simulink model "PV_GHI_System_Mezoo_3"  (R2024b)
settings: Solver=ode3  StartTime=0.0  StopTime=259200  FixedStep=60  RelTol=1e-3
InitFcn:
  | % --- تحديث كود تهيئة السيمولينك (InitFcn) ---
  | disp('>>> 1. جاري تحضير العقل (Loading Neural Network)...');
  | 
  | % تحديد المسار الصحيح للمشروع الحالي
  | Project_Path = 'D:\Project\Agent Vini';
  | if exist(Project_Path, 'dir')
  |     addpath(Project_Path);
  | end
  | 
  | % اسم الملف الجديد (تأكد أن هذا هو الاسم الموجود عندك في المجلد)
  | Model_File = 'Lightweight_Model.mat';
  | 
  | % محاولة التحميل
  | if exist(Model_File, 'file')
  |     FileData = load(Model_File);
  |     disp(['✅ تم تحميل الملف: ' Model_File]);
  | else
  |     % محاولة البحث في المجلد القديم كحل مؤقت لو الملف لم ينقل
  |     Old_Path = 'D:\Project\Agent 13';
  |     if exist(fullfile(Old_Path, 'PI_HybridNet.mat'), 'file')
  |         addpath(Old_Path);
  |         FileData = load('PI_HybridNet.mat');
  |         warning('⚠️ تم تحميل الملف القديم من Agent 13 لأن الجديد غير موجود!');
  |     else
  |         error('❌ لم يتم العثور على ملف النموذج (لا الجديد ولا القديم)!');
  |     end
  | end
  | 
  | % استخراج الشبكة (سواء كان اسمها net أو net_best أو net_light)
  | if isfield(FileData, 'net_light')
  |     net_ready = FileData.net_light;
  | elseif isfield(FileData, 'net')
  |     net_ready = FileData.net;
  | elseif isfield(FileData, 'net_best')
  |     net_ready = FileData.net_best;
  | else
  |     % ربما المتغير نفسه هو الشبكة
  |     VarNames = fieldnames(FileData);
  |     net_ready = FileData.(VarNames{1});
  | end
  | 
  | disp('>>> 2. العقل جاهز في الذاكرة باسم: net_ready');
undefined symbols (not defined in the file or in its folder): A, History_Day1, History_Day2, History_Day3, Max_Tank, mu_X, mu_Y, sig_X, sig_Y
libraries: mpclib x1
settings Model: Creator=moham  LastModifiedBy=moham
settings DebuggingCC: AlgebraicLoopMsg=none

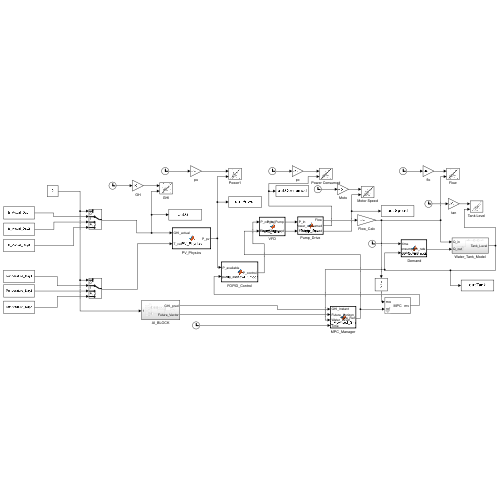
[thumbnail: Simulink's stored preview of the top-level diagram]
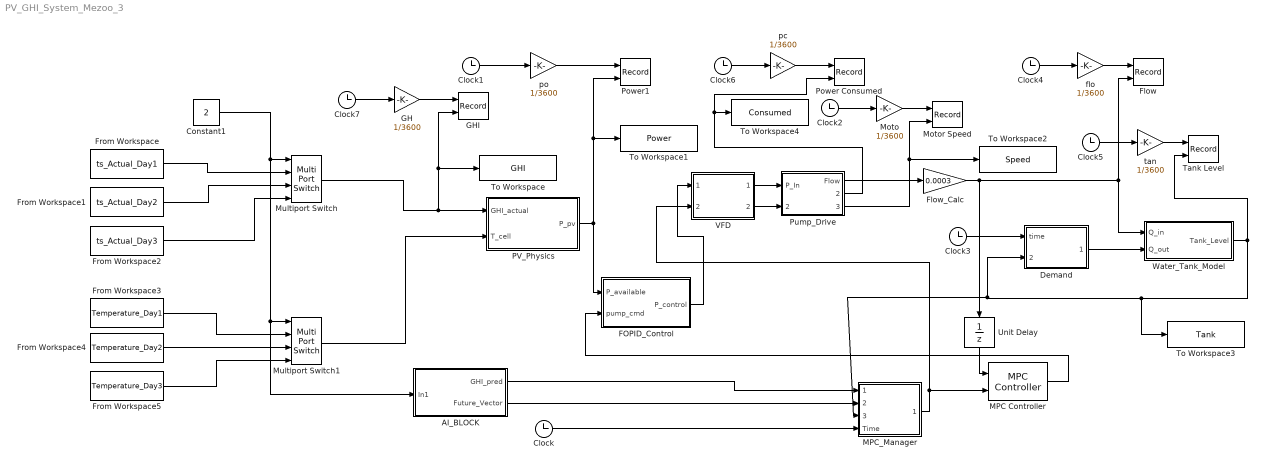
== system PV_GHI_System_Mezoo_3 ==
  " Demand" : MATLAB Function  TreatAsAtomicUnit=on
  AI_BLOCK : Subsystem
  Clock{,1..7} (8 alike) : Clock
  Constant1 : Constant  Value=2
  FOPID_Control : MATLAB Function  TreatAsAtomicUnit=on
  Flow : Record  FileSettingsInternal="{\"entries\":[{\"content\":{\"excelSettings\":{\"content\":{},\"type\":\"Streamout.ExcelSettings\"}},\"type\":\"Streamout.FileSettingStorage\",\"uuid\":\"\"}],\"packageUris\":[\"http:\\/\\/schema.mathworks.com\\/mf0\\/streamout_blocks\\/R2020a\"],\"version\":\"1.0\"}"  Layout=[1 1]  SignalsInternal="{\"entries\":[{\"content\":{\"signals\":[{\"content\":{\"blockPath\":[],\"dimensions\":[1],\"domain\":\"\",\"lineColor\":\"#b746ff\",\"lineWidth\":2,\"port\":1,\"sid\":[\"\"],\"signalID\":1,\"signalName\":\"flo\"},\"type\":\"RecordBlkView.Signal\",\"uuid\":\"\"},{\"content\":{\"blockPath\":[],\"dimensions\":[1],\"domain\":\"\",\"lineColor\":\"#64d413\",\"lineWidth\":2,\"port\":2,\"sid\":[\"\"],\"signalID\":2,\"signalName\":\"Flow_Calc\"},\"type\":\"RecordBlkView.Signal\",\"uuid\":\"\"}]},\"type\":\"RecordBlkView.InputSignals\",\"uuid\":\"\"}],\"packageUris\":[\"http:\\/\\/schema.mathworks.com\\/mf0\\/streamout_blocks\\/R2020a\"],\"version\":\"1.0\"}"  VisualizationBindings="{\"xyplotplugin\":{\"info\":[{\"series\":[],\"subplotID\":1}]}}"  CompatibilityTag=XY
  Flow_Calc : Gain  Gain=0.0003
  From Workspace : FromWorkspace  VariableName=ts_Actual_Day1
  From Workspace1 : FromWorkspace  VariableName=ts_Actual_Day2
  From Workspace2 : FromWorkspace  VariableName=ts_Actual_Day3
  From Workspace3 : FromWorkspace  VariableName=Temperature_Day1
  From Workspace4 : FromWorkspace  VariableName=Temperature_Day2
  From Workspace5 : FromWorkspace  VariableName=Temperature_Day3
  GH : Gain  Gain=1/3600
  GHI : Record  FileSettingsInternal="{\"entries\":[{\"content\":{\"excelSettings\":{\"content\":{},\"type\":\"Streamout.ExcelSettings\"}},\"type\":\"Streamout.FileSettingStorage\",\"uuid\":\"\"}],\"packageUris\":[\"http:\\/\\/schema.mathworks.com\\/mf0\\/streamout_blocks\\/R2020a\"],\"version\":\"1.0\"}"  Layout=[1 1]  SignalsInternal="{\"entries\":[{\"content\":{\"signals\":[{\"content\":{\"blockPath\":[],\"dimensions\":[1],\"domain\":\"\",\"lineColor\":\"#ff13a6\",\"lineWidth\":2,\"plots\":[ 1 ],\"port\":1,\"sid\":[\"\"],\"signalID\":1,\"signalName\":\"GH\"},\"type\":\"RecordBlkView.Signal\",\"uuid\":\"\"},{\"content\":{\"blockPath\":[],\"dimensions\":[1],\"domain\":\"\",\"lineColor\":\"#fe330a\",\"lineWidth\":2,\"plots\":[ 1 ],\"port\":2,\"sid\":[\"\"],\"signalID\":2,\"signalName\":\"Multiport\\nSwitch\"},\"type\":\"RecordBlkView.Signal\",\"uuid\":\"\"}]},\"type\":\"RecordBlkView.InputSignals\",\"uuid\":\"\"}],\"packageUris\":[\"http:\\/\\/schema.mathworks.com\\/mf0\\/streamout_blocks\\/R2020a\"],\"version\":\"1.0\"}"  VisualizationBindings="{\"xyplotplugin\":{\"info\":[{\"series\":[{\"bindingParametersList\":[{\"parameter\":\"X-Axis\",\"signalID\":1,\"signalName\":\"GH\"},{\"parameter\":\"Y-Axis\",\"signalID\":2,\"signalName\":\"Multiport\\nSwitch\"}],\"seriesID\":0}],\"subplotID\":1}]}}"  CompatibilityTag=XY
  MPC Controller : mpclib/MPC Controller  SCDEnableBlockLinearizationSpecification=on  mpcobj=MPC_Obj  is_multiple=0  enable_value=0  return_u0=off  updateMPCinCallerWorkspace=on  md_inport=off  mv_inport=off  uref_inport=off  return_cost=off  return_mvseq=off  return_qpstatus=off  return_xseq=off  return_state=off  return_ovseq=off  state_inport=off  umin_inport=off  umax_inport=off  ymin_inport=off  ymax_inport=off  cc_inport=off  ywt_inport=off  uwt_inport=off  duwt_inport=off  rhoeps_inport=off  pm_inport=off  MaximumP=10  HorizonChoice=FixedHorizon  n_ts=60  n_p=300  n_mv=1  n_md=0  n_ud=0  n_mo=1  n_uo=0  BlockDataType=double  SampleTimeInherited=off  switch_inport=off
  MPC_Manager : MATLAB Function  TreatAsAtomicUnit=on
  Moto : Gain  Gain=1/3600
  Motor Speed : Record  FileSettingsInternal="{\"entries\":[{\"content\":{\"excelSettings\":{\"content\":{},\"type\":\"Streamout.ExcelSettings\"}},\"type\":\"Streamout.FileSettingStorage\",\"uuid\":\"\"}],\"packageUris\":[\"http:\\/\\/schema.mathworks.com\\/mf0\\/streamout_blocks\\/R2020a\"],\"version\":\"1.0\"}"  Layout=[1 1]  SignalsInternal="{\"entries\":[{\"content\":{\"signals\":[{\"content\":{\"blockPath\":[],\"dimensions\":[1],\"domain\":\"\",\"lineColor\":\"#139fff\",\"lineWidth\":2,\"plots\":[ 1 ],\"port\":1,\"sid\":[\"\"],\"signalID\":1,\"signalName\":\"Moto\"},\"type\":\"RecordBlkView.Signal\",\"uuid\":\"\"},{\"content\":{\"blockPath\":[],\"dimensions\":[1],\"domain\":\"\",\"lineColor\":\"#ff6929\",\"lineWidth\":2,\"plots\":[ 1 ],\"port\":2,\"sid\":[\"\"],\"signalID\":2,\"signalName\":\"Pump_Drive:3\"},\"type\":\"RecordBlkView.Signal\",\"uuid\":\"\"}]},\"type\":\"RecordBlkView.InputSignals\",\"uuid\":\"\"}],\"packageUris\":[\"http:\\/\\/schema.mathworks.com\\/mf0\\/streamout_blocks\\/R2020a\"],\"version\":\"1.0\"}"  VisualizationBindings="{\"xyplotplugin\":{\"info\":[{\"series\":[{\"bindingParametersList\":[{\"parameter\":\"X-Axis\",\"signalID\":1,\"signalName\":\"Moto\"},{\"parameter\":\"Y-Axis\",\"signalID\":2,\"signalName\":\"Pump_Drive:3\"}],\"seriesID\":0}],\"subplotID\":1}]}}"  CompatibilityTag=XY
  Multiport Switch : MultiPortSwitch  DataPortOrder=Zero-based contiguous  DiagnosticForDefault=Warning  zeroidx=on  SaturateOnIntegerOverflow=off  InputSameDT=off
  Multiport Switch1 : MultiPortSwitch  DataPortOrder=Zero-based contiguous  DiagnosticForDefault=Warning  zeroidx=on  SaturateOnIntegerOverflow=off  InputSameDT=off
  PV_Physics : MATLAB Function  TreatAsAtomicUnit=on
  Power Consumed : Record  FileSettingsInternal="{\"entries\":[{\"content\":{\"excelSettings\":{\"content\":{},\"type\":\"Streamout.ExcelSettings\"}},\"type\":\"Streamout.FileSettingStorage\",\"uuid\":\"\"}],\"packageUris\":[\"http:\\/\\/schema.mathworks.com\\/mf0\\/streamout_blocks\\/R2020a\"],\"version\":\"1.0\"}"  Layout=[1 1]  SignalsInternal="{\"entries\":[{\"content\":{\"signals\":[{\"content\":{\"blockPath\":[],\"dimensions\":[1],\"domain\":\"\",\"lineColor\":\"#d95319\",\"lineWidth\":2,\"port\":1,\"sid\":[\"\"],\"signalID\":1,\"signalName\":\"pc\"},\"type\":\"RecordBlkView.Signal\",\"uuid\":\"\"},{\"content\":{\"blockPath\":[],\"dimensions\":[1],\"domain\":\"\",\"lineColor\":\"#edb120\",\"lineWidth\":2,\"port\":2,\"sid\":[\"\"],\"signalID\":2,\"signalName\":\"Pump_Drive:2\"},\"type\":\"RecordBlkView.Signal\",\"uuid\":\"\"}]},\"type\":\"RecordBlkView.InputSignals\",\"uuid\":\"\"}],\"packageUris\":[\"http:\\/\\/schema.mathworks.com\\/mf0\\/streamout_blocks\\/R2020a\"],\"version\":\"1.0\"}"  VisualizationBindings="{\"xyplotplugin\":{\"info\":[{\"series\":[],\"subplotID\":1}]}}"  CompatibilityTag=XY
  Power1 : Record  FileSettingsInternal="{\"entries\":[{\"content\":{\"excelSettings\":{\"content\":{},\"type\":\"Streamout.ExcelSettings\"}},\"type\":\"Streamout.FileSettingStorage\",\"uuid\":\"\"}],\"packageUris\":[\"http:\\/\\/schema.mathworks.com\\/mf0\\/streamout_blocks\\/R2020a\"],\"version\":\"1.0\"}"  Layout=[1 1]  SignalsInternal="{\"entries\":[{\"content\":{\"signals\":[{\"content\":{\"blockPath\":[],\"dimensions\":[1],\"domain\":\"\",\"lineColor\":\"#7e2f8e\",\"lineWidth\":2,\"port\":1,\"sid\":[\"\"],\"signalID\":1,\"signalName\":\"po\"},\"type\":\"RecordBlkView.Signal\",\"uuid\":\"\"},{\"content\":{\"blockPath\":[],\"dimensions\":[1],\"domain\":\"\",\"lineColor\":\"#77ac30\",\"lineWidth\":2,\"port\":2,\"sid\":[\"\"],\"signalID\":2,\"signalName\":\"PV_Physics\"},\"type\":\"RecordBlkView.Signal\",\"uuid\":\"\"}]},\"type\":\"RecordBlkView.InputSignals\",\"uuid\":\"\"}],\"packageUris\":[\"http:\\/\\/schema.mathworks.com\\/mf0\\/streamout_blocks\\/R2020a\"],\"version\":\"1.0\"}"  VisualizationBindings="{\"xyplotplugin\":{\"info\":[{\"series\":[],\"subplotID\":1}]}}"  CompatibilityTag=XY
  Pump_Drive : MATLAB Function  TreatAsAtomicUnit=on
  Tank Level : Record  FileSettingsInternal="{\"entries\":[{\"content\":{\"excelSettings\":{\"content\":{},\"type\":\"Streamout.ExcelSettings\"}},\"type\":\"Streamout.FileSettingStorage\",\"uuid\":\"\"}],\"packageUris\":[\"http:\\/\\/schema.mathworks.com\\/mf0\\/streamout_blocks\\/R2020a\"],\"version\":\"1.0\"}"  Layout=[1 1]  SignalsInternal="{\"entries\":[{\"content\":{\"signals\":[{\"content\":{\"blockPath\":[],\"dimensions\":[1],\"domain\":\"\",\"lineColor\":\"#4dbeee\",\"lineWidth\":2,\"plots\":[ 1 ],\"port\":1,\"sid\":[\"\"],\"signalID\":1,\"signalName\":\"tan\"},\"type\":\"RecordBlkView.Signal\",\"uuid\":\"\"},{\"content\":{\"blockPath\":[],\"dimensions\":[1],\"domain\":\"\",\"lineColor\":\"#a2142f\",\"lineWidth\":2,\"plots\":[ 1 ],\"port\":2,\"sid\":[\"\"],\"signalID\":2,\"signalName\":\"Water_Tank_Model\"},\"type\":\"RecordBlkView.Signal\",\"uuid\":\"\"}]},\"type\":\"RecordBlkView.InputSignals\",\"uuid\":\"\"}],\"packageUris\":[\"http:\\/\\/schema.mathworks.com\\/mf0\\/streamout_blocks\\/R2020a\"],\"version\":\"1.0\"}"  VisualizationBindings="{\"xyplotplugin\":{\"info\":[{\"series\":[{\"bindingParametersList\":[{\"parameter\":\"X-Axis\",\"signalID\":1,\"signalName\":\"tan\"},{\"parameter\":\"Y-Axis\",\"signalID\":2,\"signalName\":\"Water_Tank_Model\"}],\"seriesID\":0}],\"subplotID\":1}]}}"  CompatibilityTag=XY
  To Workspace : ToWorkspace  VariableName=GHI  SaveFormat=Timeseries  SampleTime=-1
  To Workspace1 : ToWorkspace  VariableName=Power  SaveFormat=Timeseries  SampleTime=-1
  To Workspace2 : ToWorkspace  VariableName=Speed  SaveFormat=Timeseries  SampleTime=-1
  To Workspace3 : ToWorkspace  VariableName=Tank  SaveFormat=Timeseries  SampleTime=-1
  To Workspace4 : ToWorkspace  VariableName=Consumed  SaveFormat=Timeseries  SampleTime=-1
  Unit Delay : UnitDelay  SampleTime=60  HasFrameUpgradeWarning=on
  VFD : MATLAB Function  TreatAsAtomicUnit=on
  Water_Tank_Model : Subsystem
  flo : Gain  Gain=1/3600
  pc : Gain  Gain=1/3600
  po : Gain  Gain=1/3600
  tan : Gain  Gain=1/3600
  wires:
  Water_Tank_Model/1(Tank_Level) -> To Workspace3/1, MPC_Manager/3(Water_Level), " Demand"/2(water_level), Tank Level/2
  Flow_Calc/1 -> Unit Delay/1, Flow/2, Water_Tank_Model/1(Q_in)
  Pump_Drive/1(Flow) -> Flow_Calc/1
  Pump_Drive/2(Power_consumed) -> To Workspace4/1, Power Consumed/2
  Pump_Drive/3(Motor_Speed) -> To Workspace2/1, Motor Speed/2
  Clock1/1 -> po/1
  po/1 -> Power1/1
  flo/1 -> Flow/1
  Clock4/1 -> flo/1
  Clock5/1 -> tan/1
  tan/1 -> Tank Level/1
  Clock2/1 -> Moto/1
  Moto/1 -> Motor Speed/1
  Clock6/1 -> pc/1
  pc/1 -> Power Consumed/1
  Clock7/1 -> GH/1
  GH/1 -> GHI/1
  PV_Physics/1(P_pv) -> To Workspace1/1, Power1/2, FOPID_Control/1(P_available)
  Multiport Switch/1 -> To Workspace/1, GHI/2, PV_Physics/1(GHI_actual)
  Constant1/1 -> Multiport Switch1/1, AI_BLOCK/1(In1), Multiport Switch/1
  From Workspace/1 -> Multiport Switch/2
  From Workspace1/1 -> Multiport Switch/3
  From Workspace2/1 -> Multiport Switch/4
  " Demand"/1(consumption_rate) -> Water_Tank_Model/2(Q_out)
  Clock3/1 -> " Demand"/1(time)
  FOPID_Control/1(P_control) -> VFD/1(P_control)
  VFD/1(P_to_Pump) -> Pump_Drive/1(P_In)
  VFD/2(Flow_Command) -> Pump_Drive/2(Flow_In)
  MPC_Manager/1(Flow_Ref) -> VFD/2(target_flow), MPC Controller/2
  MPC Controller/1 -> FOPID_Control/2(pump_cmd)
  Unit Delay/1 -> MPC Controller/1
  Clock/1 -> MPC_Manager/4(Time)
  AI_BLOCK/1(GHI_pred) -> MPC_Manager/1(GHI_Instant)
  From Workspace4/1 -> Multiport Switch1/3
  From Workspace3/1 -> Multiport Switch1/2
  From Workspace5/1 -> Multiport Switch1/4
  Multiport Switch1/1 -> PV_Physics/2(T_cell)
  AI_BLOCK/2(Future_Vector) -> MPC_Manager/2(Future_Horizon)

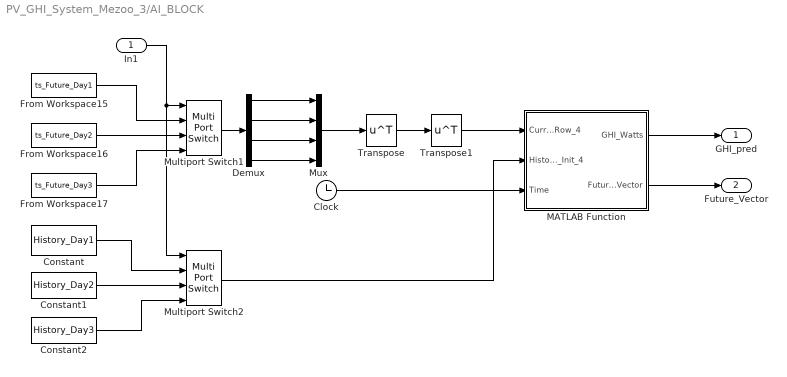
== system PV_GHI_System_Mezoo_3/AI_BLOCK ==
  In1 : Inport
  Clock : Clock
  Constant : Constant  Value=History_Day1
  Constant1 : Constant  Value=History_Day2
  Constant2 : Constant  Value=History_Day3
  Demux : Demux
  From Workspace15 : FromWorkspace  VariableName=ts_Future_Day1
  From Workspace16 : FromWorkspace  VariableName=ts_Future_Day2
  From Workspace17 : FromWorkspace  VariableName=ts_Future_Day3
  MATLAB Function : MATLAB Function  TreatAsAtomicUnit=on
  Multiport Switch1 : MultiPortSwitch  DataPortOrder=Zero-based contiguous  DiagnosticForDefault=Warning  zeroidx=on  SaturateOnIntegerOverflow=off  InputSameDT=off
  Multiport Switch2 : MultiPortSwitch  DataPortOrder=Zero-based contiguous  DiagnosticForDefault=Warning  zeroidx=on  SaturateOnIntegerOverflow=off  InputSameDT=off
  Mux : Mux
  Transpose : Math  Operator=transpose
  Transpose1 : Math  Operator=transpose
  GHI_pred : Outport
  Future_Vector : Outport  Port=2
  wires:
  From Workspace16/1 -> Multiport Switch1/3
  From Workspace17/1 -> Multiport Switch1/4
  From Workspace15/1 -> Multiport Switch1/2
  In1/1 -> Multiport Switch2/1, Multiport Switch1/1
  Multiport Switch1/1 -> Demux/1
  MATLAB Function/1(GHI_Watts) -> GHI_pred/1
  Mux/1 -> Transpose/1
  Constant/1 -> Multiport Switch2/2
  Constant1/1 -> Multiport Switch2/3
  Constant2/1 -> Multiport Switch2/4
  Multiport Switch2/1 -> MATLAB Function/2(History_Init_4)
  Transpose/1 -> Transpose1/1
  Transpose1/1 -> MATLAB Function/1(Current_Row_4)
  Clock/1 -> MATLAB Function/3(Time)
  Demux/1 -> Mux/1
  Demux/2 -> Mux/2
  Demux/3 -> Mux/3
  Demux/4 -> Mux/4
  MATLAB Function/2(Future_Vector) -> Future_Vector/1

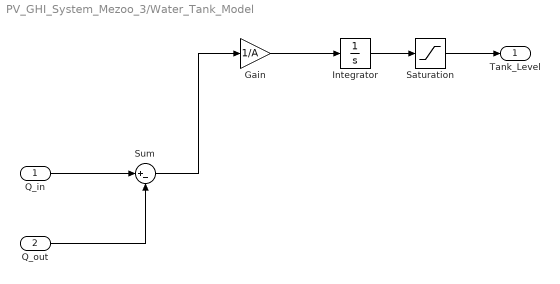
== system PV_GHI_System_Mezoo_3/Water_Tank_Model ==
  Q_in : Inport
  Q_out : Inport  Port=2
  Gain : Gain  Gain=1/A
  Integrator : Integrator  InitialCondition=4
  Saturation : Saturate  UpperLimit=Max_Tank  LowerLimit=0
  Sum : Sum  Inputs=|+-
  Tank_Level : Outport
  wires:
  Q_in/1 -> Sum/1
  Sum/1 -> Gain/1
  Integrator/1 -> Saturation/1
  Saturation/1 -> Tank_Level/1
  Q_out/1 -> Sum/2
  Gain/1 -> Integrator/1

== matlab function PV_GHI_System_Mezoo_3/FOPID_Control ==
  settings: updateMethod=DISCRETE
  data: P_available input; P_control output; pump_cmd input

function P_control = FOPID_Control_Smooth(P_available, pump_cmd)

%% FOPID Parameters (تم تنعيمها قليلاً لتقليل العدوانية)
Kp = 1.0;   % قللناها من 1.2 لتقليل رد الفعل العنيف
Ki = 0.5;   % التكامل يسبب تذبذباً إذا كان عالياً، 0.5 كافية جداً
Kd = 0.01;  % زدنا التفاضل قليلاً لامتصاص الصدمات
lambda = 0.9;
mu     = 0.7;

%% Persistent states (ذاكرة)
persistent e_int e_prev prev_P_out is_running
if isempty(e_int)
    e_int  = 0;
    e_prev = 0;
    prev_P_out = 0;   % لتنعيم الخرج
    is_running = 0;   % حالة التشغيل (للسماحية)
end

%% ===============================
%% 1. إيقاف فوري للأوامر الصفرية
%% ===============================
if pump_cmd == 0
    e_int = 0;
    e_prev = 0;
    prev_P_out = 0;
    is_running = 0;
    P_control = 0;
    return;
end

%% Reference
P_ref = pump_cmd * P_available;

%% Error definition
e = P_ref;

%% Fractional Integral
e_int = e_int + sign(e) * abs(e)^lambda;
% حماية من التراكم (Windup)
e_int = max(-5000, min(5000, e_int));

%% Fractional Derivative
de = sign(e - e_prev) * abs(e - e_prev)^mu;
e_prev = e;

%% FOPID Law
P_raw = Kp*e + Ki*e_int + Kd*de;

%% Saturation (الحدود الفيزيائية)
P_raw = max(0, min(P_available, P_raw));

%% ===============================
%% 2. نظام السماحية (Hysteresis) - مانع التذبذب رقم 1
%% ===============================
% بدلاً من رقم واحد (2200)، نستخدم رقمين:
START_THRESH = 2400;  % لا تبدأ إلا لو الطاقة قوية
STOP_THRESH  = 2000;  % لا تقف إلا لو الطاقة ضعفت جداً

if is_running == 0
    if P_raw > START_THRESH
        is_running = 1;
    else
        is_running = 0;
    end
else
    if P_raw < STOP_THRESH
        is_running = 0;
    else
        is_running = 1;
    end
end

if is_running == 0
    Target_P = 0;
    e_int = 0; % تصفير التكامل عند التوقف لمنع القفزة عند العودة
else
    Target_P = P_raw;
end

%% ===============================
%% 3. منع الصدمات (Rate Limiter) - مانع التذبذب رقم 2
%% ===============================
% نمنع الطاقة من التغير بأكثر من 100 واط في الخطوة الواحدة
% هذا يجعل صوت الموتور ناعماً ويمنع "النتعة"
MAX_RATE = 150; 

delta = Target_P - prev_P_out;

if abs(delta) > MAX_RATE
    P_control = prev_P_out + sign(delta) * MAX_RATE;
else
    P_control = Target_P;
end

% تحديث الذاكرة
prev_P_out = P_control;

end

== matlab function PV_GHI_System_Mezoo_3/ Demand ==
  data: time input; consumption_rate output; water_level input
function consumption_rate = Crop_Consumption(time, water_level)
%% =========================================================
%%  استهلاك الزراعة الواقعي (5 فدان - ري بالتنقيط - أم درمان)
%%  الاحتياج اليومي: 100,000 لتر (100 متر مكعب)
%%  نظام الري: يعمل 12 ساعة (من 6 ص إلى 6 م)
%% =========================================================

%% التوقيت
hour = mod(time/3600, 24);
DAY_START = 6; 
DAY_END = 18;

%% حساب المعدل (Base Rate)
% الهدف: 100 متر مكعب خلال 12 ساعة تشغيل
% المعادلة: 100 / (12 ساعة * 3600 ثانية) = 0.00231 m^3/s
BASE_CONSUMPTION = 0.002; 

%% منطق الاستهلاك
if (hour >= DAY_START) && (hour < DAY_END)
    % نحن في فترة النهار (ري)
    if water_level > 2.0
        % المياه متوفرة -> ري كامل
        consumption_rate = BASE_CONSUMPTION; 
    elseif water_level > 1.0
        % المياه قليلة -> تقليل الكمية للنصف
        consumption_rate = BASE_CONSUMPTION * 0.5; 
    else
        % خطر الجفاف -> إيقاف الري للحفاظ على المضخة
        consumption_rate = 0; 
    end
else
    % نحن في الليل -> لا ري
    consumption_rate = 0;
end

end

== matlab function PV_GHI_System_Mezoo_3/VFD ==
  data: P_control input; P_to_Pump output; target_flow input; Flow_Command output
function [P_to_Pump, Flow_Command] = VFD_Block(P_control, target_flow)

    %% ==========================================
    %% 1. الجزء الأصلي للـ VFD (Ramping & Jump)
    %% ==========================================
    ramp_rate_power = 5000;
    ramp_rate_flow  = 8; 
    
    persistent P_prev Flow_prev
    if isempty(P_prev), P_prev = 0; Flow_prev = 0; end
    dt = 0.01; 
    
    % --- منطق القفز الفوري للقدرة ---
    if (P_prev < 100) && (P_control > 2000)
        P_control_smooth = P_control; 
    else
        max_P_change = ramp_rate_power * dt;
        P_diff = P_control - P_prev;
        if abs(P_diff) > max_P_change
            P_control_smooth = P_prev + sign(P_diff) * max_P_change;
        else
            P_control_smooth = P_control;
        end
    end
    
    % --- منطق القفز الفوري للتدفق ---
    if (Flow_prev < 0.5) && (target_flow > 5)
        target_flow_smooth = target_flow; 
    else
        max_Flow_change = ramp_rate_flow * dt;
        Flow_diff = target_flow - Flow_prev;
        if abs(Flow_diff) > max_Flow_change
            target_flow_smooth = Flow_prev + sign(Flow_diff) * max_Flow_change;
        else
            target_flow_smooth = target_flow;
        end
    end
    
    % --- التصفير والتحديث ---
    if (P_control < 50) && (P_control_smooth < 2000)
        P_control_smooth = 0; target_flow_smooth = 0;
        P_prev = 0; Flow_prev = 0;
    else
        P_prev = P_control_smooth; Flow_prev = target_flow_smooth;
    end
    
    P_control_smooth = max(0, P_control_smooth);
    target_flow_smooth = max(0, target_flow_smooth);

    %% ==========================================
    %% 2. منطق المضخة (تم نقله هنا حرفياً) 🔻
    %% ==========================================
    
    % --- الثوابت (من كود المضخة) ---
    eta_total = 0.7;
    P_rated   = 10000;
    Flow_max  = 16;
    Speed_max = 1500;
    P_min     = 2000; % الحد الأدنى كما طلبت

    % --- الحسابات (من كود المضخة) ---
    P_useful = P_control_smooth * eta_total;
    
    if P_useful > P_min
        P_rated_hydraulic = P_rated * eta_total; 
        ratio = P_useful / P_rated_hydraulic;
        if ratio > 1; ratio = 1; end 
        
        Flow_calc = Flow_max * sqrt(ratio);
        
        % نأخذ الأقل بين المتاح والهدف
        Raw_Flow = min(target_flow_smooth, Flow_calc);
    else
        Raw_Flow = 0;
    end

    % --- حساب السرعة لفحص الشرط (من كود المضخة) ---
    if Raw_Flow > 0
        Raw_Speed = (Raw_Flow / Flow_max) * Speed_max;
    else
        Raw_Speed = 0;
    end

    % --- الفلترة الصارمة (من كود المضخة) ---
    % إذا السرعة أقل من 690، اقطع كل شيء من هنا
    if Raw_Speed < 690
        Final_Flow = 0;
        Final_P    = 0; % نقطع الكهرباء أيضاً
    else
        Final_Flow = Raw_Flow;
        Final_P    = P_control_smooth;
    end

    %% ==========================================
    %% 3. الخرج النهائي
    %% ==========================================
    P_to_Pump    = Final_P;
    Flow_Command = Final_Flow;

end

== matlab function PV_GHI_System_Mezoo_3/MPC_Manager ==
  settings: updateMethod=DISCRETE
  data: GHI_Instant input; Future_Horizon input; Flow_Ref output; Water_Level input; Time input
function Flow_Ref   = MPC_Flywheel_Smooth(GHI_Instant, Future_Horizon, Water_Level, Time)
    % =====================================================================
    % MPC FLYWHEEL SMOOTH (VELVET MODE) 🦋
    % تعديل خاص: الارتفاع رياضي وقوي، والنزول ناعم جداً "حبة حبة"
    % =====================================================================
    
    %% 1. الثوابت والبيانات
    GHI_Now = double(GHI_Instant);
    if GHI_Now < 0, GHI_Now = 0; end
    
    P_RATED = 10000; 
    AREA_PV = 60;    
    EFF_AVG = 0.16;
    
    % الحدود
    TANK_MAX_HARD = 5.3; 
    TANK_RESTART  = 4.8;  
    
    Power_Now = GHI_Now * AREA_PV * EFF_AVG;
    
    %% 2. الذاكرة
    persistent state last_switch_time Smooth_Flow
    if isempty(state)
        state = 0; 
        last_switch_time = -9999;
        Smooth_Flow = 0; 
    end
    
    elapsed = Time - last_switch_time;
    
    %% 3. المدير (القرار) 👔
    Target_Flow = 0;
    
    % [أ] منطق التشغيل/الإيقاف
    if state == 0
        % شروط التشغيل
        if (Water_Level <= TANK_RESTART) && (Power_Now > 2500) && (elapsed > 300)
            state = 1;
            last_switch_time = Time;
        end
    else 
        % شروط الإيقاف
        if (Water_Level >= TANK_MAX_HARD) || (Power_Now < 2000)
             if elapsed > 120 
                 state = 0;
                 last_switch_time = Time;
             end
        end
    end
    
    % [ب] تحديد الهدف
    if state == 1
        % حساب السرعة من الشمس
        Load_Ratio = min(1, Power_Now / P_RATED);
        Raw_Flow = 16 * (Load_Ratio)^(1/3);
        
        % الفرامل الذكية (عند الامتلاء فقط)
        Braking_Start = 17.5 - (0.5 * (Raw_Flow / 16));
        if Water_Level > Braking_Start
            Dist = TANK_MAX_HARD - Braking_Start;
            Factor = (TANK_MAX_HARD - Water_Level) / Dist;
            Factor = max(0, min(1, Factor));
            Raw_Flow = Raw_Flow * sqrt(Factor);
        end
        
        if Raw_Flow < 4.0
            Target_Flow = 0; 
        else
            Target_Flow = Raw_Flow;
        end
    else
        Target_Flow = 0;
    end
    
    %% 4. المنفذ الهيدروليكي (التعديل الجوهري هنا) 🌊✨
    % هنا السر: فرقنا بين معامل الصعود ومعامل النزول
    
    % 1. هل نحن نصعد أم ننزل؟
    if Target_Flow >= Smooth_Flow
        % --- حالة صعود (تسارع) ---
        % نخليها زي ما كانت عشان الارتفاع يكون ممتاز
        Current_Alpha = 0.08; 
    else
        % --- حالة نزول (تهدئة) ---
        % هنا طلبك: "حبة حبة وشغل ناعم"
        % صغرنا الرقم جداً (0.005) يعني المضخة حتاخد راحتها عالااااخر وهي نازلة
        % هذا يمنع الخنقة تماماً
        Current_Alpha = 0.005; 
    end
    
    % المعادلة السحرية
    Smooth_Flow = (1 - Current_Alpha) * Smooth_Flow + (Current_Alpha * Target_Flow);
    
    % تنظيف النهايات (Snap to Zero)
    % قللنا حد القطع لـ 0.1 عشان نسمح لها تنزل براحتها لحد آخر قطرة
    if Smooth_Flow < 0.1
        Smooth_Flow = 0;
    end
    
    if Smooth_Flow > 16
        Smooth_Flow = 16;
    end
    
    %% 5. الخرج النهائي
    Flow_Ref = Smooth_Flow;
    
    % حالة المضخة
    if Flow_Ref > 0.5
        Pump_State = 1;
    else
        Pump_State = 0;
    end
end

== matlab function PV_GHI_System_Mezoo_3/PV_Physics ==
  data: GHI_actual input; P_pv output; T_cell input
function P_pv = PV_Physics(GHI_actual, T_cell)
% PV_Physics
% Pure physical PV model (Updated: 590W Panel, 12kW System)
% Inputs:
%   GHI_actual : actual solar irradiance [W/m^2]
%   T_cell     : cell temperature [°C]

% --- PV Array Parameters (Updated) ---
% لكي نصل لـ 12 كيلو واط باستخدام ألواح 590 واط
% نحتاج 22 لوح تقريباً (12980 واط خام) وسيتم قصها لـ 12000
N_series   = 11;  % عدد الألواح في السلسلة الواحدة
N_parallel = 2;   % عدد السلاسل المتوازية

% --- 590W Panel Specifications (Standard Mono Perc) ---
V_mp_ref = 41.7;  % جهد الماكس
I_mp_ref = 14.15; % تيار الماكس (41.7 * 14.15 = 590 Watts)
V_oc_ref = 50.1;  % جهد الدائرة المفتوحة
I_sc_ref = 14.95; % تيار القصر

G_ref = 1000;
T_ref = 25;

% --- Temperature coefficients ---
beta_V  = -0.0031;   
alpha_I =  0.0005;   

% --- Irradiance & temperature effects ---
G_ratio = max(0, GHI_actual) / G_ref;
dT = (T_cell - T_ref);

V_mp = V_mp_ref * (1 + beta_V * dT);
I_mp = I_mp_ref * G_ratio * (1 + alpha_I * dT);

V_pv = V_mp * N_series;
I_pv = I_mp * N_parallel;

P_pv = V_pv * I_pv;

% --- Physical limits ---
V_max = V_oc_ref * N_series;
I_max = I_sc_ref * N_parallel;

V_pv = max(0, min(V_max, V_pv));
I_pv = max(0, min(I_max, I_pv));

% التحديد النهائي عند 12 كيلو واط كما طلبت
P_pv = max(0, min(12000, P_pv));   % 12 kW limit

end

== matlab function PV_GHI_System_Mezoo_3/AI_BLOCK/MATLAB Function ==
  settings: updateMethod=DISCRETE
  data: Current_Row_4 input; GHI_Watts output double size=1; History_Init_4 input; Time input; sig_Y parameter; mu_Y parameter; sig_X parameter; mu_X parameter; Future_Vector output
function [GHI_Watts, Future_Vector] = AI_Brain_Vini_4F_5H_Final(Current_Row_4, History_Init_4, Time, sig_Y, mu_Y, sig_X, mu_X)
    % =====================================================================
    % VINI BRAIN (4 FEATURES) + 5H HORIZON + LOG CORRECTION option 🌟
    % تم ضبطه ليكون آمناً تماماً مع السيمولينك (Coder Friendly)
    % ويطبق التنعيم المباشر (Direct Watt Smoothing) للدقة القصوى.
    % =====================================================================
    
    % تعريف الدوال الخارجية
    coder.extrinsic('predict');
    coder.extrinsic('evalin');
    coder.extrinsic('exist'); 
    
    % تعريف المتغيرات الدائمة
    persistent Buffer net_loaded Is_Init Last_Update_Time Target_Watts Current_Smooth_Watts Future_Preds Correction_Factor
    
    % ---------------------------------------------------------
    % 0. إعدادات التصحيح (خيارك الذكي) 📐
    % ---------------------------------------------------------
    % اجعل هذه true لتفعيل نظريتك (إضافة نصف التباين لتعويض الوسط الهندسي)
    Use_Correction = true; 
    
    % ---------------------------------------------------------
    % 1. شبكة الأمان (Safety Nets) - لضمان عدم توقف السيمولينك
    % ---------------------------------------------------------
    if isempty(Target_Watts), Target_Watts = 0; end
    if isempty(Current_Smooth_Watts), Current_Smooth_Watts = 0; end
    if isempty(Future_Preds), Future_Preds = zeros(1, 5); end
    if isempty(Last_Update_Time), Last_Update_Time = -9999; end
    if isempty(Correction_Factor), Correction_Factor = 0; end

    % ---------------------------------------------------------
    % 2. التهيئة الأولية (مرة واحدة عند التشغيل)
    % ---------------------------------------------------------
    GHI_Watts = 0;
    
    if isempty(Is_Init)
        Exists_Val = 0; 
        % محاولة تحميل النموذج الخفيف أولاً
        mx_Exists = evalin('base', "exist('Lightweight_Model.mat', 'file')");
        Exists_Val = double(mx_Exists); 
        
        if Exists_Val == 2
            net_loaded = evalin('base', 'load(''Lightweight_Model.mat'').net_light');
            % تقدير معامل التصحيح (تقريبي) إذا فعلت الخيار
            if Use_Correction, Correction_Factor = 0.005; else, Correction_Factor = 0; end
        else
            % الخيار البديل
            net_loaded = evalin('base', 'net_best'); 
            Correction_Factor = 0;
        end
        
        % تجهيز الذاكرة (24x4)
        if size(History_Init_4, 1) == 24
            Buffer = double(History_Init_4);
        else
            Buffer = double(History_Init_4');
        end
        
        Is_Init = true;
    end
    
    % قراءة القيمة الحالية للمتغير الدائم
    Future_Vector = Future_Preds;

    % ---------------------------------------------------------
    % 3. منطق التحديث (كل ساعة)
    % ---------------------------------------------------------
    Current_Hour = floor(Time / 3600);
    Last_Hour = floor(Last_Update_Time / 3600);
    
    if (Current_Hour > Last_Hour) || (Time == 0)
        
        % === [ أ. تحديث الذاكرة ] ===
        New_Feat = double(Current_Row_4(:)'); 
        Buffer(1:23, :) = Buffer(2:24, :);
        Buffer(24, :) = New_Feat;
        
        % تحضير مصفوفات التطبيع
        % انتبه: ترتيب المدخلات في الدالة هو (sig_X, mu_X)
        Mu_Mat = repmat(double(mu_X(:)'), 24, 1);
        Sig_Mat = repmat(double(sig_X(:)'), 24, 1);
        Sig_Mat(Sig_Mat == 0) = 1; 
        
        % === [ ب. التنبؤ اللحظي (Current Hour) ] ===
        Normalized_Input = (Buffer - Mu_Mat) ./ Sig_Mat;
        Net_Input = Normalized_Input'; 
        
        % حل مشكلة mxArray (الحجز المسبق)
        Val_Simple = 0; 
        mx_Output = predict(net_loaded, Net_Input, 'MiniBatchSize', 1);
        Temp_Pred_Mat = double(mx_Output);
        Val_Simple = Temp_Pred_Mat(1); 
        
        % فك التطبيع + تطبيق تصحيح اللوغاريتم (إن وجد)
        Y_Log_Val = (Val_Simple * double(sig_Y)) + double(mu_Y);
        Y_Log_Corrected = Y_Log_Val + Correction_Factor;
        
        Hour_Avg_Watts = (10^Y_Log_Corrected) - 1;
        if Hour_Avg_Watts < 0, Hour_Avg_Watts = 0; end
        
        % === [ ج. التنبؤ المستقبلي (5 ساعات) - Recursive Loop ] ===
        Temp_Buffer = Buffer;   
        Temp_Forecast = zeros(1, 5);
        Last_Pred_Norm = Val_Simple;
        
        for k = 1:5
            % 1. حساب الواط (مع التصحيح)
            Current_Y_Log = (Last_Pred_Norm * double(sig_Y)) + double(mu_Y);
            Current_Y_Corr = Current_Y_Log + Correction_Factor;
            
            Current_Pred_Watts = (10^Current_Y_Corr) - 1;
            if Current_Pred_Watts < 0, Current_Pred_Watts = 0; end
            Temp_Forecast(k) = Current_Pred_Watts;
            
            % 2. تحديث البفر للمستقبل
            Temp_Buffer(1:23, :) = Temp_Buffer(2:24, :);
            Future_Row = Temp_Buffer(23, :); 
            
            % تحديث الميزة 1 (GHI Logged) - نستخدم القيمة الخام بدون تصحيح للبفر
            Future_Row(1) = Current_Y_Log; 
            
            % الميزة 2 (CS) تبقى كما هي (Persistence)
            
            % تحديث الميزة 3 (KT) بذكاء
            CS_Val = (10^Future_Row(2)) - 1;
            if CS_Val > 5
                New_KT = Current_Pred_Watts / CS_Val;
                if New_KT > 1.2, New_KT = 1.2; end
                if New_KT < 0, New_KT = 0; end
                Future_Row(3) = New_KT;
            else
                Future_Row(3) = 0;
            end
            
            Temp_Buffer(24, :) = Future_Row;
            
            % 3. التنبؤ التالي
            Norm_Input_Fut = (Temp_Buffer - Mu_Mat) ./ Sig_Mat;
            
            Temp_Fut_Val = 0;
            mx_Fut_Out = predict(net_loaded, Norm_Input_Fut', 'MiniBatchSize', 1);
            Temp_Fut_Mat = double(mx_Fut_Out);
            Last_Pred_Norm = Temp_Fut_Mat(1);
        end
        
        % تحديث المتغيرات الدائمة
        Future_Preds = Temp_Forecast;
        Future_Vector = Future_Preds;

        % === [ د. تحديد الهدف (Watt Smoothing) ] ===
        % الهدف هو القيمة المباشرة وليس نسبة
        Target_Watts = Hour_Avg_Watts;
        
        % في اللحظة صفر، نبدأ من الهدف مباشرة
        if Time == 0
            Current_Smooth_Watts = Target_Watts;
        end
        
        Last_Update_Time = Time;
    end
    
    % ---------------------------------------------------------
    % 4. التنعيم المباشر (Direct Watt Smoothing) 🌊
    % ---------------------------------------------------------
    % هذا الفلتر يضمن انسيابية المنحنى ومطابقته لدقة الأفق
    Alpha = 0.04; % معامل نعومة متوسط (يمكنك تغييره لـ 0.02 لنعومة أكبر)
    
    Current_Smooth_Watts = (1 - Alpha) * Current_Smooth_Watts + (Alpha * Target_Watts);
    
    GHI_Watts = Current_Smooth_Watts;
    if GHI_Watts < 0, GHI_Watts = 0; end
end

== matlab function PV_GHI_System_Mezoo_3/Pump_Drive ==
  data: P_In input; Flow_In input; Flow output; Power_consumed output; Motor_Speed output
function [Flow, Power_consumed, Motor_Speed] = Pump_Drive(P_In, Flow_In)

    % 1. تمرير القيم الجاهزة من الـ VFD
    Flow = Flow_In;
    Power_consumed = P_In;

    % 2. حساب السرعة (للرسم فقط)
    % نفس المعادلة: Speed = (Flow / 16) * 1500
    if Flow > 0
        Motor_Speed = (Flow / 16.0) * 1550;
    else
        Motor_Speed = 0;
    end
    
    % حماية الرسم (Saturate)
    Motor_Speed = max(0, min(1550, Motor_Speed));

end
